simulink model "rtwdemo_udt"  (Simulink 7.6)
settings: Solver=FixedStepDiscrete  StartTime=0.0  StopTime=10  FixedStep=1  RelTol=1e-3  SampleTimeConstraint=STIndependent
PostLoadFcn:
  | rtwdemo_udt_data
libraries: rtwdemowidgets x1
Description:
  | User-Defined Data Type Objects to Define Numeric Types and Aliases
settings Model: Creator=The MathWorks Inc.  ExtModeAutoUpdateStatusClock=off
settings DataIOCC: SaveOutput=off  SaveTime=off  SignalLoggingName=logsOut
settings OptimizationCC: InlineParams=on  InlineInvariantSignals=on  PassReuseOutputArgsAs=Individual arguments  StateBitsets=on  DataBitsets=on  UseTempVars=on  ZeroExternalMemoryAtStartup=off  ZeroInternalMemoryAtStartup=off  NoFixptDivByZeroProtection=on  EfficientFloat2IntCast=on  EfficientMapNaN2IntZero=off  OptimizeModelRefInitCode=on  LifeSpan=1  BufferReusableBoundary=off
settings DebuggingCC: CheckExecutionContextPreStartOutputMsg=on  CheckExecutionContextRuntimeOutputMsg=on  SolverPrmCheckMsg=none  StrictBusMsg=ErrorOnBusTreatedAsVector
settings HardwareCC: ProdIntDivRoundTo=Zero  ProdEndianess=LittleEndian  ProdHWDeviceType=Generic->32-bit Embedded Processor  TargetHWDeviceType=Generic->32-bit Embedded Processor
settings ModelReferenceCC: UpdateModelReferenceTargets=IfOutOfDate
settings SFSimCC: SimParseCustomCode=off
settings RTWCC: SystemTargetFile=ert.tlc  TLCOptions=-p0 -aWarnNonSaturatedBlocks=0  TemplateMakefile=ert_default_tmf  Description=Real-Time Workshop Embedded Coder (no auto configuration)  GenerateReport=on  RTWVerbose=off  ProcessScript=ert_make_rtw_hook  IncludeHyperlinkInReport=on  LaunchReport=on
settings CodeAppCC: ForceParamTrailComments=on  IgnoreCustomStorageClasses=off  IgnoreTestpoints=on  SimulinkDataObjDesc=on  CustomSymbolStrFcn=$N$M$F  CustomSymbolStrMacro=$N$M  InsertBlockDesc=on
settings ERTTargetCC: TargetFcnLib=ansi_tfl_tmw.mat  MultiwordLength=2048  GenerateSampleERTMain=on  IncludeMdlTerminateFcn=off  SupportNonFinite=off  SupportComplex=off  InlinedParameterPlacement=NonHierarchical  ERTCustomFileTemplate=example_file_process.tlc  ConvertIfToSwitch=off  EnableUserReplacementTypes=on
settings MATStruct: double=FLOAT64  single=FLOAT32  int32=S32  int16=S16  int8=S8  uint32=U32  uint16=U16  uint8=U8  boolean=U8  int=S32  uint=U32  char=CHAR

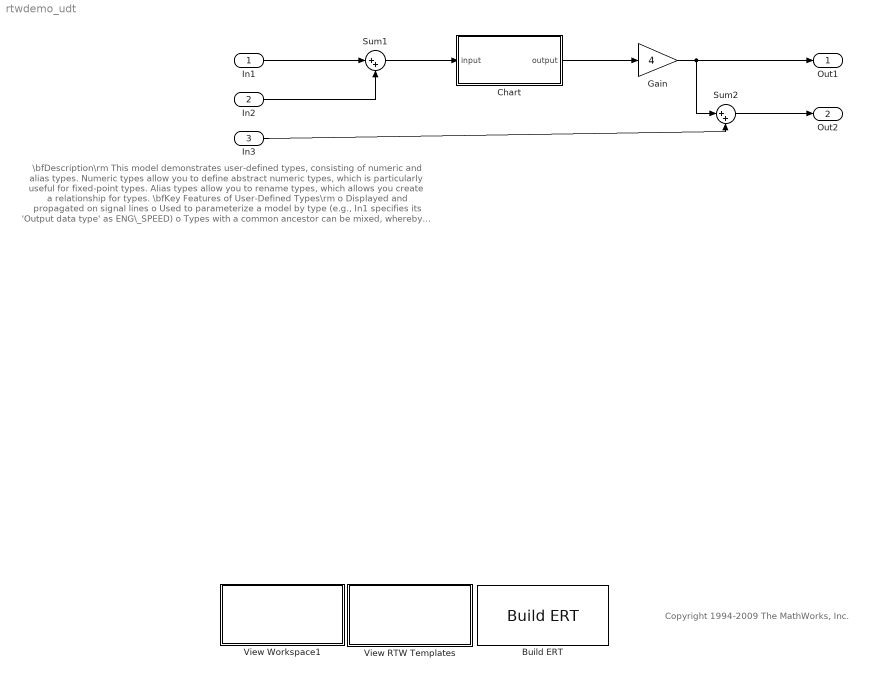
== system rtwdemo_udt ==
  note: \bfDescription\rm
      | This model demonstrates user-defined types, consisting of numeric and alias types.  Numeric types allow you
      | to define abstract numeric types, which is particularly useful for fixed-point types.  Alias types allow you to rename
      | types, which allows you create a relationship for types.
      |
      | \bfKey Features of User-Defined Types\rm
      | o Displayed and propagated on signal lines
      | o Used to parameterize a model by type (e.g., In1 specifies its 'Output data type' as ENG\_SPEED)
      | o Types with a common ancestor can be mixed, whereby the common ancestor is propagated (e.g., output of Sum1)
      | o Intrinsically supported by the Simulink Model Explorer
      | o Include an optional header file attribute that is ideal for importing legacy types (ignored for GRT targets)
      | o Types used in the generated code (ignored for GRT targets)
      |
      | \bfInstructions\rm
      | 1. Inspect the user-defined types in the Model Explorer by double-clicking the first yellow button below.
      | 2. Inspect the replacement data type mapping by double-clicking the second yellow button below.
      | 3. Compile the diagram to display the types in this model (Edit > Update Diagram or Ctrl+B).
      | 4. Generate code with the blue button below and inspect model files to see how user-defined types
      |     appear in the generated code.
      | 5. Modify the attributes of ENG\_SPEED and ENG\_SPEED\_OFFSET and repeat steps 1-4.
      |
      | \bfNotes\rm
      | o User-defined types are a feature of Simulink that facilitate parameterization of the data types in a model.
      |    Real-Time Workshop Embedded Coder preserves alias data type names (e.g., ENG\_SPEED) in the generated
      |    code, whereas Real-Time Workshop implements user-define types as their base type (e.g., real32\_T).
      | o Real-Time Workshop Embedded Coder also enables you to replace the built-in data types with user-defined
      |    data types in the generated code.
  note: Copyright 1994-2009 The MathWorks, Inc.
  In1 : Inport  OutDataTypeStr=ENG_SPEED  PortDimensions=1
  In2 : Inport  Port=2  OutDataTypeStr=ENG_SPEED_OFFSET  PortDimensions=1
  In3 : Inport  Port=3  OutDataTypeStr=int16  PortDimensions=1
  Build ERT : rtwdemowidgets/Build ERT  SystemSampleTime=-1  attrib_overrides={'EnableUserReplacementTypes', 'ReplacementTypes'}
  Chart : Stateflow chart  TreatAsAtomicUnit=on
  Gain : Gain  Gain=4  OutDataTypeStr=ENG_SPEED
  Sum1 : Sum  Inputs=|++
  Sum2 : Sum  Inputs=|++
  View RTW Templates : Subsystem
      settings: OpenFcn=|
      | dlg = slCfgPrmDlg(bdroot,'Open');
      | dlg = slCfgPrmDlg(bdroot,'TurnToPage','Real-Time Workshop/Data Type Replacement'); clear dlg;
      mask Display: disp('View Data Type\nReplacements\n(double-click)')
  View Workspace1 : Subsystem
      settings: OpenFcn=rtwprivate daexplrwsview;
      mask Display: disp('View Data\nType Objects\n(double-click)')
  Out1 : Outport
  Out2 : Outport  Port=2
  wires:
  In2/1 -> Sum1/2
  In1/1 -> Sum1/1
  Sum1/1 -> Chart/1(input)
  Gain/1 -> Out1/1, Sum2/1
  In3/1 -> Sum2/2
  Sum2/1 -> Out2/1
  Chart/1(output) -> Gain/1

== system rtwdemo_udt/View RTW Templates ==

== system rtwdemo_udt/View Workspace1 ==

== stateflow chart Chart ==
  (default) -> (junction 3)
  (junction 3) -> (junction 4) [order 1] : [input > 5]
      |   {output = 5 + (input-5)/2;}
  (junction 3) -> (junction 4) [order 2] : {output = input;}
  data: input input ENG_SPEED; output output ENG_SPEED
